simulink model "Single_media_filtration"  (Simulink 7.9)
settings: Solver=ode15s  SolverMode=SingleTasking  StartTime=0.0  StopTime=6*24*3600  RelTol=1e-5  AbsTol=1e-5
undefined symbols (not defined in the file): B, U, x0
settings Model: Creator=psross  LastModifiedBy=M.Sparnaaij  ExtModeTrigMode=oneshot  ExtModeArmWhenConnect=off
settings DataIOCC: LimitDataPoints=off  SaveOutput=off  SaveTime=off  SignalLoggingName=sigsOut
settings OptimizationCC: BooleanDataType=off
settings DebuggingCC: SaveWithParameterizedLinksMsg=none  SignalResolutionControl=TryResolveAllWithWarning  SolverPrmCheckMsg=none  MultiTaskDSMMsg=warning  MultiTaskCondExecSysMsg=none  FcnCallInpInsideContextMsg=Use local settings  StrictBusMsg=None
settings HardwareCC: TargetUnknown=on
settings RTWCC: IncludeERTFirstTime=on
settings GRTTargetCC: CombineOutputUpdateFcns=off  GRTInterface=on

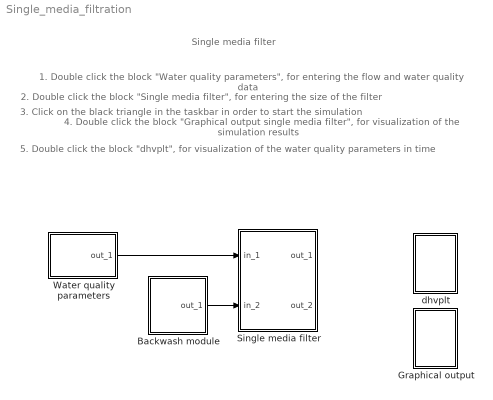
== system Single_media_filtration ==
  note: Single media filter
  note: 2. Double click the block "Single media filter", for entering the size of the filter
  note: 3. Click on the black triangle in the taskbar in order to start the simulation
  note: 4. Double click the block "Graphical output single media filter", for visualization of the simulation results
  note: 1. Double click the block "Water quality parameters", for entering the flow and water quality data
  note: 5. Double click the block "dhvplt", for visualization of the water quality parameters in time
  Backwash module : Subsystem  Description=During a simulation the filter can be backwashed with the backwash module, so a number of successive filterruns can be simulated.
      mask init:
      | filenaam='./StimelaData/Backwash_module.mat';
      | 
      | [Pn,Fn,Fext]=Fileprop(filenaam);
      | 
      | errstr = st_UniqName(filenaam,'filenaam=''','SubSystem','OpenFcn');
      | if errstr, error([errstr 'The filename "' filenaam '" is already in use. Choose a different filename.']), end
      | 
      | P = bacwa1_p(filenaam);
      | [B,x0,U]=bacwa1_i(filenaam);
      settings: OpenFcn=|
      | filenaam='./StimelaData/Backwash_module.mat';
      | st_ParameterInput('init',gcb,filenaam,'bacwa1');
      mask Display:
      | plot(0,0,100,100,[80,80,20,20],[80,20,20,80],[40,42,38,40,40],[70,67,67,70,30],[60,62,58,60,60],[70,67,67,70,30]);
      | disp('')
      | text(50,50,'bacwa1', 'horizontalAlignment', 'center', 'verticalAlignment', 'middle');
      | text(50,0,Fn, 'horizontalAlignment', 'center', 'verticalAlignment', 'base');
  Graphical output : Subsystem
      settings: OpenFcn=enkfil_g
      mask Display:
      | plot(0,0,100,100,[80,20,20],[20,20,80],[80,69,60,52,45,39,33,28,24,20],[65,65,64,61,57,52,45,37,30,20])
      | disp('');
      | text(100,100,'enkfil', 'horizontalAlignment', 'right', 'verticalAlignment', 'top');
  Single media filter : Subsystem  Description=This model calculates the removal of suspended solids with a single media filter.
      mask init:
      | filenaam='./StimelaData/Single_media_filter.mat';
      | 
      | [Pn,Fn,Fext]=Fileprop(filenaam);
      | 
      | errstr = st_UniqName(filenaam,'filenaam=''','SubSystem','OpenFcn');
      | if errstr, error([errstr 'The filename "' filenaam '" is already in use. Choose a different filename.']), end
      | 
      | P = enkfil_p(filenaam);
      | [B,x0,U]=enkfil_i(filenaam);
      settings: OpenFcn=|
      | filenaam='./StimelaData/Single_media_filter.mat';
      | st_ParameterInput('init',gcb,filenaam,'enkfil');
      mask Display:
      | plot(0,0,100,100,[25.000000,25.000000,75.000000,75.000000,87.500000],[75.000000,25.000000,25.000000,30.000000,30.000000],[87.500000,75.000000,75.000000],[37.500000,37.500000,75.000000],[25.000000,75.000000],[65.000000,65.000000],[25.000000,75.000000],[42.500000,42.500000],[37.500000,42.500000],[52.500000,52.500000],[50.000000,55.000000],[52.500000,52.500000],[62.500000,67.500000],[52.500000,52.500000])
      | disp('')
      | text(50,50,'enkfil', 'horizontalAlignment', 'center', 'verticalAlignment', 'middle');
      | text(50,0,Fn, 'horizontalAlignment', 'center', 'verticalAlignment', 'base');
  Water quality parameters : Subsystem  Description=The water flow and the water quality data must be filled out in the 'Water quality parameters' block. Each project must start with a 'Water quality parameters' block.
      mask init:
      | filenaam='./StimelaData/Water_qual_param.mat';
      | 
      | [Pn,Fn,Fext]=Fileprop(filenaam);
      | 
      | errstr = st_UniqName(filenaam,'filenaam=''','SubSystem','OpenFcn');
      | if errstr, error([errstr 'The filename "' filenaam '" is already in use. Choose a different filename.']), end
      | 
      | P = invruw_p(filenaam);
      | [B,x0,U]=invruw_i(filenaam);
      settings: OpenFcn=|
      | filenaam='./StimelaData/Water_qual_param.mat';
      | st_ParameterInput('init',gcb,filenaam,'invruw');
      mask Display:
      | plot(0,0,100,100,[80 100],[ 50 50],[80 100],[ 55 55],[20 80 80 20 20],[10 10 90  90 10]);
      | disp('')
      | text(50,50,'invruw', 'horizontalAlignment', 'center', 'verticalAlignment', 'middle');
      | text(50,0,Fn, 'horizontalAlignment', 'center', 'verticalAlignment', 'base');
  dhvplt : Subsystem
      settings: OpenFcn=plotStimela2
      mask Display:
      | plot(0,0,100,100,[80,20,20],[20,20,80],[80,69,60,52,45,39,33,28,24,20],[65,65,64,61,57,52,45,37,30,20])
      | disp('');
      | text(100,100,'Stimela', 'horizontalAlignment', 'right', 'verticalAlignment', 'top');
  wires:
  Water quality parameters/1(out_1) -> Single media filter/1(in_1)
  Backwash module/1(out_1) -> Single media filter/2(in_2)

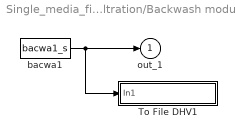
== system Single_media_filtration/Backwash module ==
  To File DHV1 : Subsystem  mask(To File DHV){naam=[filenaam(1:length(filenaam)-4) '_out.sti']}
      mask prompts: naam "Naam van bestand"
      mask init:
      | set_param([gcb '/To File'],'Filename',naam);
      mask Display: disp(naam)
  bacwa1 : S-Function  FunctionName=bacwa1_s  Parameters=B,x0,U,P  EnableBusSupport=off
  out_1 : Outport  InitialOutput=0
  wires:
  bacwa1/1 -> out_1/1, To File DHV1/1(In1)

== system Single_media_filtration/Graphical output ==
  note: plotten

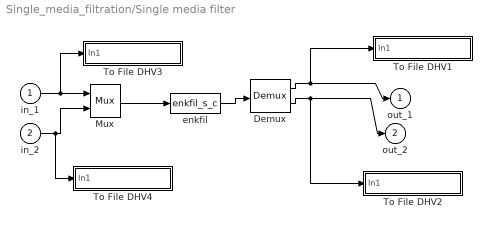
== system Single_media_filtration/Single media filter ==
  in_1 : Inport
  in_2 : Inport  Port=2
  Demux : Demux  Outputs=[U.Number B.Measurements]
  Mux : Mux  Inputs=[U.Number B.Setpoints]
  To File DHV1 : Subsystem  mask(To File DHV){naam=[filenaam(1:length(filenaam)-4) '_out.sti']}
      mask prompts: naam "Naam van bestand"
      mask init:
      | set_param([gcb '/To File'],'Filename',naam);
      mask Display: disp(naam)
  To File DHV2 : Subsystem  mask(To File DHV){naam=[filenaam(1:length(filenaam)-4) '_EM.sti']}
      mask prompts: naam "Naam van bestand"
      mask init:
      | set_param([gcb '/To File'],'Filename',naam);
      mask Display: disp(naam)
  To File DHV3 : Subsystem  mask(To File DHV){naam=[filenaam(1:length(filenaam)-4) '_in.sti']}
      mask prompts: naam "Naam van bestand"
      mask init:
      | set_param([gcb '/To File'],'Filename',naam);
      mask Display: disp(naam)
  To File DHV4 : Subsystem  mask(To File DHV){naam=[filenaam(1:length(filenaam)-4) '_ES.sti']}
      mask prompts: naam "Naam van bestand"
      mask init:
      | set_param([gcb '/To File'],'Filename',naam);
      mask Display: disp(naam)
  enkfil : S-Function  FunctionName=enkfil_s_c  Parameters=B,x0,U,P  EnableBusSupport=off
  out_1 : Outport  InitialOutput=0
  out_2 : Outport  Port=2  InitialOutput=0
  wires:
  Demux/2 -> out_2/1, To File DHV2/1(In1)
  Demux/1 -> out_1/1, To File DHV1/1(In1)
  enkfil/1 -> Demux/1
  in_1/1 -> Mux/1, To File DHV3/1(In1)
  Mux/1 -> enkfil/1
  in_2/1 -> Mux/2, To File DHV4/1(In1)

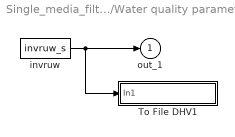
== system Single_media_filtration/Water quality parameters ==
  To File DHV1 : Subsystem  mask(To File DHV){naam=[filenaam(1:length(filenaam)-4) '_out.sti']}
      mask prompts: naam "Naam van bestand"
      mask init:
      | set_param([gcb '/To File'],'Filename',naam);
      mask Display: disp(naam)
  invruw : S-Function  FunctionName=invruw_s  Parameters=B,x0,U,P  EnableBusSupport=off
  out_1 : Outport  InitialOutput=0
  wires:
  invruw/1 -> out_1/1, To File DHV1/1(In1)

== system Single_media_filtration/dhvplt ==
  note: plotten

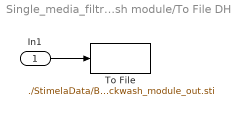
== system Single_media_filtration/Backwash module/To File DHV1 ==
  In1 : Inport
  To File : ToFile  Filename=./StimelaData/Backwash_module_out.sti  MatrixName=bacwa1out
  wires:
  In1/1 -> To File/1

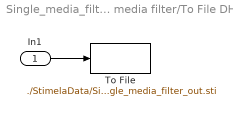
== system Single_media_filtration/Single media filter/To File DHV1 ==
  In1 : Inport
  To File : ToFile  Filename=./StimelaData/Single_media_filter_out.sti  MatrixName=enkfilout
  wires:
  In1/1 -> To File/1

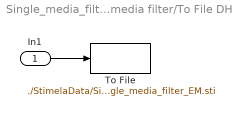
== system Single_media_filtration/Single media filter/To File DHV2 ==
  In1 : Inport
  To File : ToFile  Filename=./StimelaData/Single_media_filter_EM.sti  MatrixName=enkfilEM
  wires:
  In1/1 -> To File/1

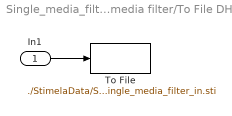
== system Single_media_filtration/Single media filter/To File DHV3 ==
  In1 : Inport
  To File : ToFile  Filename=./StimelaData/Single_media_filter_in.sti  MatrixName=enkfilin
  wires:
  In1/1 -> To File/1

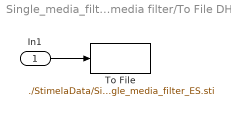
== system Single_media_filtration/Single media filter/To File DHV4 ==
  In1 : Inport
  To File : ToFile  Filename=./StimelaData/Single_media_filter_ES.sti  MatrixName=enkfilES
  wires:
  In1/1 -> To File/1

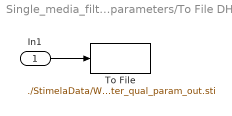
== system Single_media_filtration/Water quality parameters/To File DHV1 ==
  In1 : Inport
  To File : ToFile  Filename=./StimelaData/Water_qual_param_out.sti  MatrixName=invruwout
  wires:
  In1/1 -> To File/1
